simulink model "BothOptimized4"  (R2024b)
settings: Solver=FixedStepAuto  StartTime=0.0  StopTime=10.0  RelTol=1e-3  EnableMultiTasking=on
undefined symbols (not defined in the file or in its folder): samplingTime
settings Model: STM32="{\"DigitalPortWrite\":[{\"ID\":\"MicroMouseTemplate:84:3\"},{\"ID\":\"MicroMouseTemplate:84:4\"},{\"ID\":\"MicroMouseTemplate:84:5\"},{\"ID\":\"MicroMouseTemplate:84:6\"},{\"ID\":\"MicroMouseTemplate:84:7\"},{\"ID\":\"MicroMouseTemplate:84:8\"},{\"ID\":\"MicroMouseTemplate:84:9\"},{\"ID\":\"MicroMouseTemplate:84:10\"},{\"ID\":\"MicroMouseTemplate:160:19\"},{\"ID\":\"MicroMouseTemplate:2479:4\"},{\"ID\":\"MicroMouseTemplate:2479:6\"},{\"ID\":\"MicroMouseTemplate:2479:7\"},{\"ID\":\"MicroMouseTemplate:2479:8\"},{\"ID\":\"MicroMouseTemplate2:160:19\"},{\"ID\":\"MicroMouseTemplate2:2479:4\"},{\"ID\":\"MicroMouseTemplate2:2479:6\"},{\"ID\":\"MicroMouseTemplate2:2479:7\"},{\"ID\":\"MicroMouseTemplate2:2479:8\"},{\"ID\":\"MicroMouseTemplate2:84:3\"},{\"ID\":\"MicroMouseTemplate2:84:4\"},{\"ID\":\"MicroMouseTemplate2:84:5\"},{\"ID\":\"MicroMouseTemplate2:84:6\"},{\"ID\":\"MicroMouseTemplate2:84:7\"},{\"ID\":\"MicroMouseTemplate2:84:8\"},{\"ID\":\"MicroMouseTemplate2:84:9\"},{\"ID\":\"MicroMouseTemplate2:84:10\"},{\"ID\":\"MicroMouseTemplateTest:160:19\"},{\"ID\":\"MicroMouseTemplateTest:2479:4\"},{\"ID\":\"MicroMouseTemplateTest:2479:6\"},{\"ID\":\"MicroMouseTemplateTest:2479:7\"},{\"ID\":\"MicroMouseTemplateTest:2479:8\"},{\"ID\":\"MicroMouseTemplateTest:84:3\"},{\"ID\":\"MicroMouseTemplateTest:84:4\"},{\"ID\":\"MicroMouseTemplateTest:84:5\"},{\"ID\":\"MicroMouseTemplateTest:84:6\"},{\"ID\":\"MicroMouseTemplateTest:84:7\"},{\"ID\":\"MicroMouseTemplateTest:84:8\"},{\"ID\":\"MicroMouseTemplateTest:84:9\"},{\"ID\":\"MicroMouseTemplateTest:84:10\"},{\"ID\":\"MicroMouseTemplateTest2:160:19\"},{\"ID\":\"MicroMouseTemplateTest2:2479:4\"},{\"ID\":\"MicroMouseTemplateTest2:2479:6\"},{\"ID\":\"MicroMouseTemplateTest2:2479:7\"},{\"ID\":\"MicroMouseTemplateTest2:2479:8\"},{\"ID\":\"MicroMouseTemplateTest2:84:3\"},{\"ID\":\"MicroMouseTemplateTest2:84:4\"},{\"ID\":\"MicroMouseTemplateTest2:84:5\"},{\"ID\":\"MicroMouseTemplateTest2:84:6\"},{\"ID\":\"MicroMouseTemplateTest2:84:7\"},{\"ID\":\"MicroMouseTemplateTest2:84:8\"},{\"ID\":\"MicroMouseTemplateTest2:84:9\"},{\"ID\":\"MicroMouseTemplateTest2:84:10\"},{\"ID\":\"HalfOptimized:84:10\"},{\"ID\":\"HalfOptimized:84:9\"},{\"ID\":\"HalfOptimized:84:8\"},{\"ID\":\"HalfOptimized:84:7\"},{\"ID\":\"HalfOptimized:84:6\"},{\"ID\":\"HalfOptimized:84:5\"},{\"ID\":\"HalfOptimized:84:4\"},{\"ID\":\"HalfOptimized:84:3\"},{\"ID\":\"HalfOptimized:160:19\"},{\"ID\":\"HalfOptimized:2479:4\"},{\"ID\":\"HalfOptimized:2479:6\"},{\"ID\":\"HalfOptimized:2479:7\"},{\"ID\":\"HalfOptimized:2479:8\"},{\"ID\":\"HalfOptimized4:84:3\"},{\"ID\":\"HalfOptimized4:84:4\"},{\"ID\":\"HalfOptimized4:84:5\"},{\"ID\":\"HalfOptimized4:84:6\"},{\"ID\":\"HalfOptimized4:84:7\"},{\"ID\":\"HalfOptimized4:84:8\"},{\"ID\":\"HalfOptimized4:84:9\"},{\"ID\":\"HalfOptimized4:84:10\"},{\"ID\":\"HalfOptimized4:160:19\"},{\"ID\":\"HalfOptimized4:2479:4\"},{\"ID\":\"HalfOptimized4:2479:6\"},{\"ID\":\"HalfOptimized4:2479:7\"},{\"ID\":\"HalfOptimized4:2479:8\"},{\"ID\":\"LeftOptimized4:84:3\"},{\"ID\":\"LeftOptimized4:84:4\"},{\"ID\":\"LeftOptimized4:84:5\"},{\"ID\":\"LeftOptimized4:84:6\"},{\"ID\":\"LeftOptimized4:84:7\"},{\"ID\":\"LeftOptimized4:84:8\"},{\"ID\":\"LeftOptimized4:84:9\"},{\"ID\":\"LeftOptimized4:84:10\"},{\"ID\":\"LeftOptimized4:160:19\"},{\"ID\":\"LeftOptimized4:2479:4\"},{\"ID\":\"LeftOptimized4:2479:6\"},{\"ID\":\"LeftOptimized4:2479:7\"},{\"ID\":\"LeftOptimized4:2479:8\"}],\"PWMOutput\":[{\"ID\":\"MicroMouseTemplate:160:24\"},{\"ID\":\"MicroMouseTemplate:160:25\"},{\"ID\":\"MicroMouseTemplate2:160:24\"},{\"ID\":\"MicroMouseTemplate2:160:25\"},{\"ID\":\"MicroMouseTemplateTest:160:24\"},{\"ID\":\"MicroMouseTemplateTest:160:25\"},{\"ID\":\"MicroMouseTemplateTest2:160:24\"},{\"ID\":\"MicroMouseTemplateTest2:160:25\"},{\"ID\":\"HalfOptimized:160:24\"},{\"ID\":\"HalfOptimized:160:25\"},{\"ID\":\"HalfOptimized4:160:24\"},{\"ID\":\"HalfOptimized4:160:25\"},{\"ID\":\"LeftOptimized4:160:24\"},{\"ID\":\"LeftOptimized4:160:25\"}],\"AnalogInput\":[{\"ID\":\"MicroMouseTemplate:2357:1\"},{\"ID\":\"MicroMouseTemplate2:2357:1\"},{\"ID\":\"MicroMouseTemplateTest:2357:1\"},{\"ID\":\"MicroMouseTemplateTest2:2357:1\"},{\"ID\":\"HalfOptimized:2357:1\"},{\"ID\":\"HalfOptimized4:2357:1\"},{\"ID\":\"LeftOptimized4:2357:1\"}],\"DigitalPortRead\":[{\"ID\":\"MicroMouseTemplate:2483:3\"},{\"ID\":\"MicroMouseTemplate:2483:4\"},{\"ID\":\"MicroMouseTemplate2:2483:3\"},{\"ID\":\"MicroMouseTemplate2:2483:4\"},{\"ID\":\"MicroMouseTemplateTest:2483:3\"},{\"ID\":\"MicroMouseTemplateTest:2483:4\"},{\"ID\":\"MicroMouseTemplateTest2:2483:3\"},{\"ID\":\"MicroMouseTemplateTest2:2483:4\"},{\"ID\":\"HalfOptimized:2483:3\"},{\"ID\":\"HalfOptimized:2483:4\"},{\"ID\":\"HalfOptimized4:2483:3\"},{\"ID\":\"HalfOptimized4:2483:4\"},{\"ID\":\"LeftOptimized4:2483:3\"},{\"ID\":\"LeftOptimized4:2483:4\"}]}"  SimulationMode=external  ExtModeTrigDuration=10  Creator=JesseJabezArendse  LastModifiedBy=Nang'alelwa
settings SolverCC: AllowMultiTaskInputOutput=on  AutoInsertRateTranBlk=on  InsertRTBMode=Never (minimum delay)
settings OptimizationCC: EnhancedBackFolding=on  PassReuseOutputArgsAs=Individual arguments  StateBitsets=on  DataBitsets=on  ZeroExternalMemoryAtStartup=off  ZeroInternalMemoryAtStartup=off  NoFixptDivByZeroProtection=on  MaxStackSize=64  OptimizeBlockOrder=speed  DifferentSizesBufferReuse=on  EfficientTunableParamExpr=on
settings DebuggingCC: MultiTaskCondExecSysMsg=none  ParameterOverflowMsg=none  ParameterPrecisionLossMsg=none  ParameterTunabilityLossMsg=error
settings HardwareCC: ProdBitPerPointer=32  ProdBitPerSizeT=32  ProdBitPerPtrDiffT=32  ProdLargestAtomicInteger=Long  ProdLargestAtomicFloat=Double  ProdWordSize=32  ProdLongLongMode=on  ProdHWDeviceType=ARM Compatible->ARM Cortex  TargetBitPerPointer=64  TargetBitPerSizeT=64  TargetBitPerPtrDiffT=64  TargetLongLongMode=on  TargetIntDivRoundTo=Zero  TargetEndianess=LittleEndian  TargetWordSize=64  TargetHWDeviceType=MATLAB Host
settings ModelReferenceCC: EnableParallelModelReferenceBuilds=on  ParallelModelReferenceMATLABWorkerInit=Copy Base Workspace  SupportModelReferenceSimTargetCustomCode=on
settings SFSimCC: MATLABDynamicMemAlloc=off  SimHardwareAcceleration=native
settings RTWCC: Description=Embedded Coder  SystemTargetFile=ert.tlc  HardwareBoard=STM32L4xx Based  TLCOptions=-p0 -aInlineSetEventsForThisBaseRateFcn=TLC_FALSE -aSuppressMultiTaskScheduler=TLC_FALSE -aRateBasedStepFcn=1  TemplateMakefile=ert_default_tmf  Toolchain=GNU Tools for ARM Embedded Processors  CodeExecutionProfiling=on  CodeProfilingInstrumentation=coarse  GPUComputeCapability=3.5
settings RTWCC: CustomHeaderCode=|
  | #include "MicroMouseProgramming\Core\Inc\IMU.h"
  | #include "MicroMouseProgramming\Core\Inc\CustomWhile.h"
  | #include "MicroMouseProgramming\Core\Inc\Motors.h"
settings RTWCC: CustomInclude=|
  | MicroMouseProgramming\Core\Inc\
  | MicroMouseProgramming\Core\Src\
settings RTWCC: CustomSource=|
  | MicroMouseProgramming\Core\Src\IMU.c
  | MicroMouseProgramming\Core\Src\CustomWhile.c
  | MicroMouseProgramming\Core\Src\Motors.c
settings CodeAppCC: ForceParamTrailComments=on  IgnoreCustomStorageClasses=off  OperatorAnnotations=on  SimulinkDataObjDesc=on  SFDataObjDesc=on  InsertBlockDesc=on
settings ERTTargetCC: CodeReplacementLibrary=ARM Cortex-M  SupportNonFinite=off  SupportComplex=off  ExtModeTransport=3  ExtModeStaticAlloc=on  ExtModeStaticAllocSize=2048  ExtModeMexFile=ext_xcp  ExtModeIntrfLevel=Level2 - Open  InlinedParameterPlacement=Hierarchical  DynamicArrayContainerType=coder::array

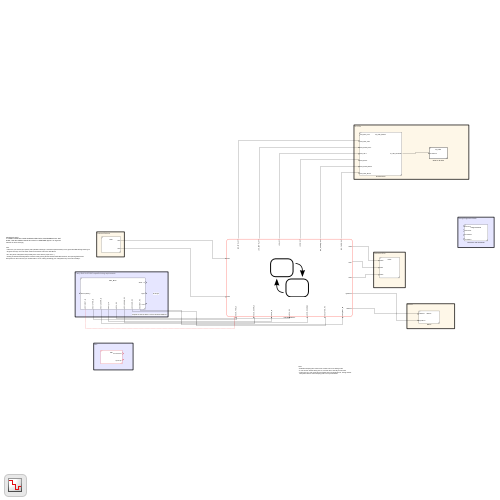
[thumbnail: Simulink's stored preview of the top-level diagram]
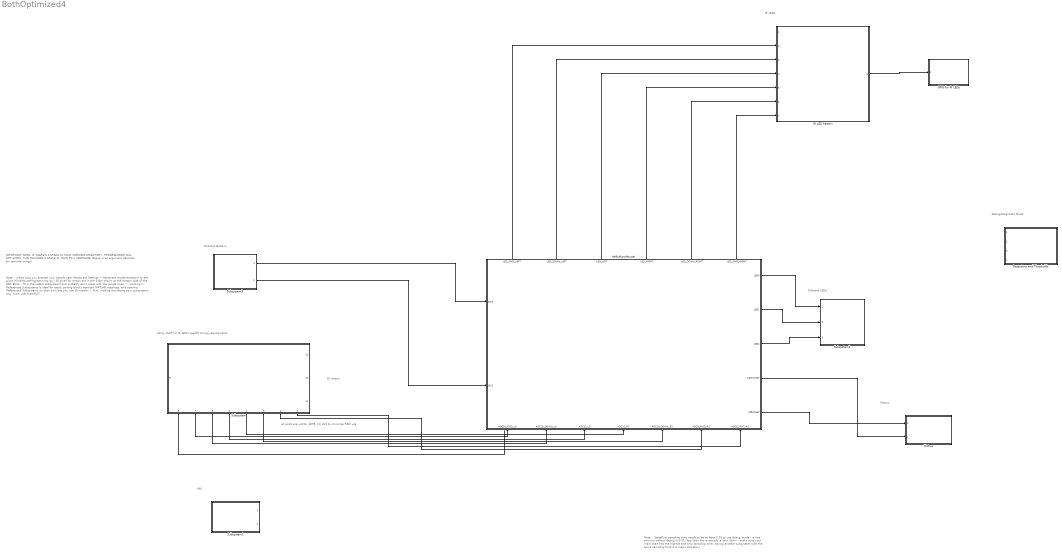
== system BothOptimized4 ==
  note: IMPORTANT NOTE:
      | IF THERE'S A SPACE IN YOUR WORKING DIRECTORY, PROGRAMMING WILL NOT WORK, THIS INCLUDES A SPACE IN YOUR PC's USERNAME (Space is an argument delimiter for terminal things)
  note: Note:
      | - make sure you entered your specifc path (Hardware Settings > Hardware Implementation) to the given MicroMouseProgramming.ioc
      | - All given 8x arrays are in the order shown at the bottom side of the ADC Block
      |
      | - fill in the yellow subsystems and probably don't mess with the purple ones :)
      | - working in Referenced Subsystems is ideal for easily porting blocks between MATLAB instances, and opening Referenced Subsystems on their own lets you use Simulation > Run, making simulating your subsystems way more user friendly!!!
  note: 8x arrays
  note: all ports are uint16, 4095 == 3V3 to minimize RAM use
  note: IMU
  note: Note:
      | - Stateflow sampling time needs to be at least 0.05 to use debug mode
      | - a nice amount without debug is 0.01, less than this is actually a slow down
      | - make sure your main chart has the highest and only sampling time, having another
      | subsystem with the same sampling time is a major slowdown
  note: Fancy Stuff for IR ADCs specific timing requirements
  note: IR LEDs
  note: Motors
  note: Onboard Buttons
  note: Onboard LEDs
  note: Debug/Diagnostic Mode
  Detections and Thresholds : Subsystem  ReferencedSubsystem=DiagnosticMode
  GPIO for IR LEDs : Subsystem  TreatAsAtomicUnit=on  SystemSampleTime=samplingTime  ReferencedSubsystem=IR_LEDs
  HelloMicroMouse! : Stateflow chart  TreatAsAtomicUnit=on
      settings: PortSchema="{\"entries\":[{\"content\":{\"sides\":[{\"content\":{\"connectorIds\":[\"In9\",\"In8\"]},\"type\":\"ConnectorPlacement.EquallySpacedRectSide\",\"uuid\":\"f52daa4f-6374-42e5-9ef1-0ccc99d09b58\"},{\"content\":{\"connectorIds\":[\"Out11\",\"Out5\",\"Out6\",\"Out2\",\"Out1\"],\"side\":\"RIGHT\"},\"type\":\"ConnectorPlacement.EquallySpacedRectSide\",\"uuid\":\"94b478cc-4dde-45c7-a588-77cf2b43cdb7\"},{\"content\":{\"connectorIds\":[\"Out3\",\"Out4\",\"Out7\",\"Out8\",\"Out9\",\"Out10\"],\"side\":\"TOP\"},\"type\":\"ConnectorPlacement.EquallySpacedRectSide\",\"uuid\":\"afff2079-ea5c-423e-9722-09c3bbce433b\"},{\"content\":{\"connectorIds\":[\"In1\",\"In2\",\"In3\",\"In4\",\"In5\",\"In6\",\"In7\"],\"side\":\"BOTTOM\"},\"type\":\"ConnectorPlacement.EquallySpacedRectSide\",\"uuid\":\"94e93a1d-795d-41a3-b2d8-d520b2bf47ef\"}]},\"type\":\"ConnectorPlacement.EquallySpacedConnector\",\"uuid\":\"d4d35636-54af-48ac-af70-d56caef5e090\"}],\"packageUris\":[\"http://schema.mathworks.com/mf0/Connector/R2020b\"],\"version\":\"1.0\"}"
  IR LED Pattern : Subsystem  ReferencedSubsystem=IR_LED_Pattern
  Motors : Subsystem  ReferencedSubsystem=Motors
      settings: PortSchema="{\"entries\":[{\"content\":{\"sides\":[{\"content\":{\"connectorIds\":[\"In2\",\"In1\"]},\"type\":\"ConnectorPlacement.EquallySpacedRectSide\",\"uuid\":\"b3741f01-871a-479c-9206-f0581f668097\"},{\"content\":{\"side\":\"RIGHT\"},\"type\":\"ConnectorPlacement.EquallySpacedRectSide\",\"uuid\":\"4e24163a-f10e-40fa-a35f-86add3e4876d\"},{\"content\":{\"side\":\"TOP\"},\"type\":\"ConnectorPlacement.EquallySpacedRectSide\",\"uuid\":\"20b900cb-8f31-42f3-9ac1-0d679ccd8bc0\"}]},\"type\":\"ConnectorPlacement.EquallySpacedConnector\",\"uuid\":\"90358f46-f7a9-48cf-9149-c68081c17f53\"}],\"packageUris\":[\"http://schema.mathworks.com/mf0/Connector/R2020b\"],\"version\":\"1.0\"}"
  Subsystem : Subsystem  ReferencedSubsystem=ADC_Block
      settings: PortSchema="{\"entries\":[{\"content\":{\"sides\":[{\"content\":{},\"type\":\"ConnectorPlacement.EquallySpacedRectSide\",\"uuid\":\"be6b81d5-7a49-4e34-b35f-0c07892094fc\"},{\"content\":{\"connectorIds\":[\"Out1\",\"Out2\",\"Out3\",\"Out4\",\"Out5\",\"Out6\",\"Out7\",\"Out8\"],\"side\":\"RIGHT\"},\"type\":\"ConnectorPlacement.EquallySpacedRectSide\",\"uuid\":\"5e22590a-b7c0-4c63-8de4-8d81fd6c3849\"},{\"content\":{\"connectorIds\":[\"Out12\",\"Out10\",\"Out11\"],\"side\":\"TOP\"},\"type\":\"ConnectorPlacement.EquallySpacedRectSide\",\"uuid\":\"da97636e-cea0-4a10-8fe5-d807f9ee999f\"},{\"content\":{\"connectorIds\":[\"Out9\"],\"side\":\"BOTTOM\"},\"type\":\"ConnectorPlacement.EquallySpacedRectSide\",\"uuid\":\"a593d780-81a8-4730-a8bc-2bbf356cafe4\"}]},\"type\":\"ConnectorPlacement.EquallySpacedConnector\",\"uuid\":\"0bcac921-e51a-4437-9183-315712d0a8c2\"}],\"packageUris\":[\"http://schema.mathworks.com/mf0/Connector/R2020b\"],\"version\":\"1.0\"}"
  Subsystem1 : Subsystem  ReferencedSubsystem=IMU
  Subsystem2 : Subsystem  ReferencedSubsystem=LEDs
  Subsystem3 : Subsystem  ReferencedSubsystem=SWs
  wires:
  HelloMicroMouse!/2(rightWheel) -> Motors/1
  HelloMicroMouse!/1(leftWheel) -> Motors/2
  IR LED Pattern/1 -> GPIO for IR LEDs/1
  Subsystem3/1 -> HelloMicroMouse!/9(SW1)
  Subsystem3/2 -> HelloMicroMouse!/8(SW2)
  HelloMicroMouse!/11(LED0) -> Subsystem2/1
  Subsystem/8 -> ?
  Subsystem/7 -> HelloMicroMouse!/1(ADC14_FWD_LS)
  Subsystem/6 -> HelloMicroMouse!/2(ADC13_DOWN_LS)
  Subsystem/5 -> HelloMicroMouse!/3(ADC12_LS)
  Subsystem/4 -> HelloMicroMouse!/4(ADC11_RS)
  Subsystem/3 -> HelloMicroMouse!/5(ADC10_DOWN_RS)
  Subsystem/2 -> HelloMicroMouse!/6(ADC9_FWD_RS)
  Subsystem/1 -> HelloMicroMouse!/7(ADC8_MOT_RS)
  HelloMicroMouse!/5(LED1) -> Subsystem2/2
  HelloMicroMouse!/6(LED2) -> Subsystem2/3
  HelloMicroMouse!/10(LED_FWD_RIGHT) -> IR LED Pattern/7
  HelloMicroMouse!/9(LED_DOWN_RIGHT) -> IR LED Pattern/6
  HelloMicroMouse!/8(LED_RIGHT) -> IR LED Pattern/5
  HelloMicroMouse!/7(LED_LEFT) -> IR LED Pattern/4
  HelloMicroMouse!/4(LED_DOWN_LEFT) -> IR LED Pattern/3
  HelloMicroMouse!/3(LED_FWD_LEFT) -> IR LED Pattern/2

== stateflow chart BothOptimized4/HelloMicroMouse! ==
  state ButtonPressed6 [commented out]
    entry:
    LED0 = false;
    LED1 = false;
    LED2 = false;
    state Turning_Right_Adjustment [commented out]
      entry:
      LED2 = true;
      leftWheel = 75;
      rightWheel = 70;
      exit:
      leftWheel = 0;
      LED2 = false;
    state Forward [commented out]
      entry:
      LED1 = true;
      % if abs(ADC13_DOWN_LS - ADC10_DOWN_RS) > down_error
      %    error = true;
      %    check = max(ADC13_DOWN_LS - thresh_down_l, ADC10_DOWN_RS - thresh_down_r)
      %end
      leftWheel = normal_speed_LEFT;
      rightWheel = normal_speed_RIGHT;
      exit:
      LED1 = false;
      % during:
      % curr_d_left = ADC13_DOWN_LS;
      % curr_d_right = ADC10_DOWN_RS;
      % if abs(curr_d_left - curr_d_right) > down_error
      %     error = true;
      %    check = max((curr_d_left - thresh_down_l)*0.8, curr_d_right - thresh_down_r)
      % end
    state Turning_Left_Adjustment [commented out]
      entry:
      LED0 = true;
      rightWheel = 75;
      leftWheel = 70;
      exit:
      rightWheel = 0;
      LED0 = false;
    (default) -> ButtonPressed6.Forward [commented out]
    ButtonPressed6.Forward -> ButtonPressed6.Turning_Right_Adjustment [commented out] : [(ADC13_DOWN_LS > thresh_DOWN_LEFT) ]
    ButtonPressed6.Turning_Right_Adjustment -> ButtonPressed6.Forward [commented out] : after(0.2, sec)
    ButtonPressed6.Forward -> ButtonPressed6.Turning_Left_Adjustment [commented out] : [(ADC10_DOWN_RS > thresh_DOWN_RIGHT) ]
    ButtonPressed6.Turning_Left_Adjustment -> ButtonPressed6.Forward [commented out] : after(0.2, sec)
  state Turns1
    entry:
    solved = 0
    LED0 = false;
    LED1 = false;
    LED2 = false;
    R = 1;
    S = 2;
    L = 3;
    B = 4;
    stop = 0
    state TurnLeftToLeft1
      entry:
      leftWheel = -75;
      rightWheel = 75;
    state CheckLeftWall1
      entry:
      leftWheel = 0;
      rightWheel = 0;
      if (ADC14_FWD_LS >0.85* init_FWD_LEFT &&  ADC9_FWD_RS >0.85* init_FWD_RIGHT)
      LED1 = false;
      else
      SolvedAlgorithm(index) = L;
      index = index +1;
      stop = 1
      LED1 = true;
      end
    state MoveCentre
      entry:
      leftWheel = 75;
      rightWheel = 75;
    state CheckStraightWall
      entry:
      leftWheel = 0;
      rightWheel = 0;
      if (ADC14_FWD_LS >0.85* init_FWD_LEFT &&  ADC9_FWD_RS >0.8* init_FWD_RIGHT)
      LED1 = false;
      else
      SolvedAlgorithm(index) = S;
      index = index +1;
      stop = 1;
      LED1 = true;
      end
    state TurnRightToStraight
      entry:
      leftWheel = 75;
      rightWheel = -75;
    state CheckLeftWall
      entry:
      leftWheel = 0;
      rightWheel = 0;
      if (ADC14_FWD_LS >0.80* init_FWD_LEFT &&  ADC9_FWD_RS >0.85* init_FWD_RIGHT)
      LED1 = false;
      else
      SolvedAlgorithm(index) = R;
      index = index +1;
      stop = 1
      LED1 = true;
      end
    state TurnRightToRight
      entry:
      leftWheel = 75;
      rightWheel = -75;
    state CheckWallBack
      entry:
      leftWheel = 0;
      rightWheel = 0;
      during:
      if (ADC14_FWD_LS >0.85* init_FWD_LEFT &&  ADC9_FWD_RS >0.87* init_FWD_RIGHT)
      LED1 = false;
      else
      SolvedAlgorithm(index) = B;
      index = index +1;
      stop = 1
      LED1 = true;
      end
    state TurnLeftToBack
      entry:
      leftWheel = 75;
      rightWheel = -75;
    (default) -> Turns1.MoveCentre
    Turns1.CheckWallBack -> TurnLeftToLeft1 : [SW2]
    TurnLeftToLeft1 -> CheckLeftWall1 : after(1.2, sec)
    Turns1.MoveCentre -> TurnLeftToLeft1 : after(0.4,sec)
    CheckLeftWall1 -> TurnRightToStraight : after(1.2,sec)
    TurnRightToStraight -> Turns1.CheckStraightWall : after(1.2,sec)
    Turns1.CheckStraightWall -> Turns1.TurnRightToRight : after(1.1,sec)
    Turns1.TurnRightToRight -> Turns1.CheckLeftWall : after(1.2,sec)
    Turns1.CheckLeftWall -> Turns1.TurnLeftToBack : after(1.2,sec)
    Turns1.TurnLeftToBack -> Turns1.CheckWallBack : after(1.2 ,sec)
  state ButtonPressed8 [commented out]
    entry:
    LED0 = false;
    LED1 = false;
    LED2 = false;
    state Driving [commented out]
      % State: Waiting
      entry:
      timer = 0;
      during:
      timer = timer + 1;
      % Transition Condition
      [timer >= 100]
      state Straight [commented out]
        entry:
        leftWheel = 75;
        rightWheel = 75;
        LED0 =false;
        LED2 = false;
        LED1 = false;
      state TurnLeft [commented out]
        entry:
        leftWheel = 75;
        rightWheel = 85;
        LED0 = true;
        LED2 = false;
        LED1 = false;
      state TurnRight [commented out]
        entry:
        rightWheel = 75;
        leftWheel = 85;
        LED2 = true;
        LED0 =false;
        LED1 =false;
      (default) -> Straight [commented out]
      Straight -> ButtonPressed8.Driving.TurnRight [commented out] : [ADC13_DOWN_LS>thresh_DOWN_LEFT]
      Straight -> ButtonPressed8.Driving.TurnLeft [commented out] : [ADC10_DOWN_RS > thresh_DOWN_RIGHT]
      ButtonPressed8.Driving.TurnLeft -> Straight [commented out] : [ADC10_DOWN_RS < thresh_DOWN_RIGHT && ADC13_DOWN_LS<thresh_DOWN_LEFT ]
      ButtonPressed8.Driving.TurnRight -> Straight [commented out] : [ADC10_DOWN_RS < thresh_DOWN_RIGHT && ADC13_DOWN_LS<thresh_DOWN_LEFT]
      ButtonPressed8.Driving.TurnRight -> ButtonPressed8.Driving.TurnLeft [commented out] : [ADC10_DOWN_RS > thresh_DOWN_RIGHT]
      ButtonPressed8.Driving.TurnLeft -> ButtonPressed8.Driving.TurnRight [commented out] : [ADC13_DOWN_LS>thresh_DOWN_LEFT]
    state FrontDetection [commented out]
      entry:
      leftWheel = 0;
      rightWheel = 0;
      LED0 =false;
      LED1 = true;
      LED2 = false;
    state CrossDetection [commented out]
      entry:
      flag = 1;
      leftWheel = 0;
      rightWheel = 0;
      LED0 =true;
      LED1 = true;
      LED2 = true;
    (default) -> Driving [commented out]
    Driving -> FrontDetection [commented out] : [averageFront > frontThreshold]
    FrontDetection -> Driving [commented out] : [averageFront< frontThreshold]
    Driving -> CrossDetection [commented out] : [averageDown < crossThreshold && timer >= 100]
    CrossDetection -> Driving [commented out] : [after(1000, msec)]{LED1 = false;}
  state Calibration_Down3 [commented out]
    entry:
    LED1 = true
    LED_FWD_LEFT = true;
    LED_FWD_RIGHT = true;
    LED_DOWN_RIGHT = true;
    LED_DOWN_LEFT = true;
    rightWheel = 75;
    leftWheel = -75;
    DOWN_R_DARK = ADC10_DOWN_RS;
    DOWN_L_DARK = ADC13_DOWN_LS;
    DOWN_R_LIGHT = ADC10_DOWN_RS;
    DOWN_L_LIGHT = ADC13_DOWN_LS;
    during:
    DOWN_R_DARK = min(DOWN_R_DARK, ADC10_DOWN_RS);
    DOWN_L_DARK = min(DOWN_L_DARK, ADC13_DOWN_LS);
    DOWN_R_LIGHT = max(DOWN_R_LIGHT, ADC10_DOWN_RS);
    DOWN_L_LIGHT = max(DOWN_L_LIGHT, ADC13_DOWN_LS);
  state Calibration_Forward3 [commented out]
    entry:
    LED1 = true;
    LED_FWD_LEFT = true;
    LED_FWD_RIGHT = true;
    LED_DOWN_RIGHT = true;
    LED_DOWN_LEFT = true;
    counter = 0
    sum_FWD_LEFT = 0;
    sum_FWD_RIGHT = 0;
    during:
    % Collect ADC values for averaging
    if counter < 100
    sum_FWD_LEFT = sum_FWD_LEFT + ADC14_FWD_LS;
    sum_FWD_RIGHT = sum_FWD_RIGHT + ADC9_FWD_RS;
    counter = counter + 1;
    else
    % Once 10 samples are collected, calculate the average
    avg_FWD_LEFT = sum_FWD_LEFT / counter;
    avg_FWD_RIGHT = sum_FWD_RIGHT / counter;
    % Use the averages for calibration or further processing
    init_FWD_LEFT = avg_FWD_LEFT;
    init_FWD_RIGHT = avg_FWD_RIGHT;
    end
  state Stop8 [commented out]
    entry:
    LED0 = false;
    LED2 = false;
    leftWheel = 0;
    rightWheel = 0;
    during:
    LED1 = ~LED1;
  state Ready4 [commented out]
    entry:
    rightWheel = 0;
    leftWheel = 0;
    LED2 = true;
    LED0 = true;
    %thresh_DOWN_RIGHT = init_DOWN_R_DARK*1.5
    %thresh_DOWN_LEFT = init_DOWN_L_DARK*1.5
    thresh_DOWN_RIGHT = (DOWN_R_LIGHT + DOWN_R_DARK)*0.5;
    thresh_DOWN_LEFT = (DOWN_L_LIGHT + DOWN_L_DARK)*0.5;
    % down_error = abs(dark_val_r - dark_val_l);
    normal_speed_LEFT = 75;
    normal_speed_RIGHT = 75;
  state WaitUntilButtonPressed10 [commented out]
    entry:
    LED_MOT_LEFT = false;
    LED_MOT_RIGHT = false;
    LED_FWD_LEFT = false;
    LED_FWD_RIGHT = false;
    LED_LEFT = false;
    LED_RIGHT = false;
    LED_DOWN_RIGHT = false;
    LED_DOWN_LEFT = false;
    during:
    LED1 = ~LED1;
  state Turns [commented out]
    entry:
    solved = 0
    LED0 = false;
    LED1 = false;
    LED2 = false;
    R = 1;
    S = 2;
    L = 3;
    B = 4;
    state TurnRightToRight [commented out]
      entry:
      leftWheel = 75;
      rightWheel = -75;
    state CheckRightWall [commented out]
      entry:
      leftWheel = 0;
      rightWheel = 0;
      if (ADC14_FWD_LS >0.85* init_FWD_LEFT &&  ADC9_FWD_RS >0.85* init_FWD_RIGHT)
      LED1 = false;
      else
      SolvedAlgorithm(index) = R;
      index = index +1;
      LED1 = true;
      end
    state MoveCentre [commented out]
      entry:
      leftWheel = 75;
      rightWheel = 75;
    state CheckStraightWall [commented out]
      entry:
      leftWheel = 0;
      rightWheel = 0;
      if (ADC14_FWD_LS >0.85* init_FWD_LEFT &&  ADC9_FWD_RS >0.85* init_FWD_RIGHT)
      LED1 = false;
      else
      SolvedAlgorithm(index) = S;
      index = index +1;
      LED1 = true;
      end
    state TurnLeftToStraight [commented out]
      entry:
      leftWheel = -75;
      rightWheel = 75;
    state CheckLeftWall [commented out]
      entry:
      leftWheel = 0;
      rightWheel = 0;
      if (ADC14_FWD_LS >0.85* init_FWD_LEFT &&  ADC9_FWD_RS >0.85* init_FWD_RIGHT)
      LED1 = false;
      else
      SolvedAlgorithm(index) = L;
      index = index +1;
      LED1 = true;
      end
    state TurnLeftToLeft [commented out]
      entry:
      leftWheel = -75;
      rightWheel = 75;
    state CheckWallBack [commented out]
      entry:
      leftWheel = 0;
      rightWheel = 0;
      during:
      if (ADC14_FWD_LS >0.85* init_FWD_LEFT &&  ADC9_FWD_RS >0.85* init_FWD_RIGHT)
      LED1 = false;
      else
      SolvedAlgorithm(index) = B;
      index = index +1;
      LED1 = true;
      end
    state TurnLeftToBack [commented out]
      entry:
      leftWheel = -75;
      rightWheel = 75;
    (default) -> Turns.MoveCentre [commented out]
    Turns.CheckWallBack -> Turns.TurnRightToRight [commented out] : [SW2]
    Turns.TurnRightToRight -> CheckRightWall [commented out] : after(1.05, sec)
    Turns.MoveCentre -> Turns.TurnRightToRight [commented out] : after(0.4,sec)
    CheckRightWall -> TurnLeftToStraight [commented out] : after(1.1,sec)
    TurnLeftToStraight -> Turns.CheckStraightWall [commented out] : after(1.2,sec)
    Turns.CheckStraightWall -> TurnLeftToLeft [commented out] : after(1.1,sec)
    TurnLeftToLeft -> Turns.CheckLeftWall [commented out] : after(1.2,sec)
    Turns.CheckLeftWall -> Turns.TurnLeftToBack [commented out] : after(1.1,sec)
    Turns.TurnLeftToBack -> Turns.CheckWallBack [commented out] : after(1.2 ,sec)
  state Placeholder2
    entry:
    index = 1;
    leftWheel = 0;
    rightWheel = 0;
    solved = 1;
    during:
    LED1=~LED1;
  state ButtonPressed7 [commented out]
    entry:
    LED1 = false;
    LED0 = false;
    LED2 = false;
    state Check_Front [commented out]
      entry:
      leftWheel = 0;
      rightWheel = 0;
      LED1 = ~LED1;
      LED0 = false;
      LED2 = ~LED2;
      during:
      LED1 = ~LED1;
      LED0 = false;
      LED2 = ~LED2;
    state Reverse [commented out]
      entry:
      leftWheel = -75;
      rightWheel = -75;
    state Turn_Around [commented out]
      entry:
      leftWheel = -motor_speed_left;
      rightWheel = motor_speed_right;
      during:
      LED1 = ~LED1;
      LED0 = ~LED0;
      LED2 = ~LED2;
    state Off_Left [commented out]
      entry:
      LED0 = true;
      leftWheel = 75;
      rightWheel = 70;
      exit:
      leftWheel = 0;
      LED0 = false;
    state Forward [commented out]
      entry:
      LED1 = false;
      LED0 = false;
      LED2 = false;
      LED_FWD_RIGHT = 1;
      LED_FWD_LEFT = 1;
      LED_RIGHT = 0;
      LED_LEFT = 0;
      leftWheel = motor_speed_left;
      rightWheel = motor_speed_right;
    state Off_Right [commented out]
      entry:
      LED2 = true;
      rightWheel = 75;
      leftWheel = 70;
      exit:
      rightWheel = 0;
      LED2 = false;
    state Check_Right [commented out]
      entry:
      LED1 = true;
      %ambient_RIGHT = ADC11_RS;
      %ambient_LEFT = ADC12_LS;
      LED_FWD_RIGHT = 0;
      LED_FWD_LEFT = 0;
      LED_RIGHT = 1;
      LED_LEFT = 1;
      leftWheel = 0;
      rightWheel = 0;
    state Turn_Right [commented out]
      entry:
      leftWheel = motor_speed_left;
      rightWheel = -motor_speed_right;
      LED_FWD_RIGHT = 1;
      LED_FWD_LEFT = 1;
      LED_RIGHT = 0;
      LED_LEFT = 0;
      LED1 = true;
      LED0 = true;
      LED2 = true;
    state Checking [commented out]
      during:
      LED1 = ~LED1
      %right_dif = abs(ADC11_RS - ambient_RIGHT);
      %left_dif = abs(ADC12_LS - ambient_LEFT);
      exit:
      LED1 = true;
    state Waiting [commented out]
      entry:
      leftWheel = motor_speed_left;
      rightWheel = motor_speed_right;
      LED1 = true;
      LED0 = true;
      LED2 = true;
    Turn_Around -> (junction 373) [commented out] : after(1.2, sec)
    (junction 373) -> Check_Front [commented out] : [ADC10_DOWN_RS >= thresh_down_r*1.15 && ADC10_DOWN_RS > thresh_down_r*1.15]
    Reverse -> Turn_Around [commented out] : [ADC13_DOWN_LS <= dark_val_l*1.15 && ADC10_DOWN_RS <= dark_val_r*1.15]
    Check_Front -> Turn_Around [commented out] : [ADC14_FWD_LS > init_FWD_LEFT || ADC9_FWD_RS > init_FWD_RIGHT]
    Reverse -> Turn_Around [commented out] : after(1,sec)
    ButtonPressed7.Forward -> Reverse [commented out] : [ADC14_FWD_LS > init_FWD_LEFT &&  ADC9_FWD_RS > init_FWD_RIGHT]
    Check_Front -> ButtonPressed7.Forward [commented out] : [ADC14_FWD_LS <= init_FWD_LEFT ||  ADC9_FWD_RS <= init_FWD_RIGHT]
    (junction 368) -> Off_Left [commented out] : [(ADC13_DOWN_LS - thresh_down_l) > (ADC10_DOWN_RS - thresh_down_r)]
    (default) -> ButtonPressed7.Forward [commented out]
    ButtonPressed7.Forward -> Off_Left [commented out] : [ADC13_DOWN_LS > thresh_down_l]
    Off_Left -> ButtonPressed7.Forward [commented out] : after(0.2, sec)
    ButtonPressed7.Forward -> Off_Right [commented out] : [ADC10_DOWN_RS > thresh_down_r]
    Off_Right -> ButtonPressed7.Forward [commented out] : after(0.2, sec)
    ButtonPressed7.Forward -> Check_Right [commented out] : [ADC13_DOWN_LS <= dark_val_l*1.15 && ADC10_DOWN_RS <= dark_val_r*1.15]
    (junction 364) -> ButtonPressed7.Forward [commented out] : [ADC10_DOWN_RS <= thresh_down_r*1.15 && ADC13_DOWN_LS <= thresh_down_l*1.15]
    ButtonPressed7.Forward -> (junction 368) [commented out] : [ADC13_DOWN_LS > thresh_down_l && ADC10_DOWN_RS > thresh_down_r]
    (junction 368) -> Off_Right [commented out] : [(ADC13_DOWN_LS - thresh_down_l) < (ADC10_DOWN_RS - thresh_down_r)]
    Turn_Right -> (junction 364) [commented out] : after(0.8, sec)
    Check_Right -> Checking [commented out] : after(0.2, sec)
    Waiting -> Turn_Right [commented out] : after(0.5, sec)
    Checking -> Waiting [commented out] : after(0.3, sec)
  state Stop7 [commented out]
    entry:
    LED_FWD_LEFT = 0;
    LED_FWD_RIGHT = 0;
    LED_LEFT = 1;
    LED_RIGHT = 1;
    LED0 = false;
    LED2 = false;
    leftWheel = 0;
    rightWheel = 0;
    during:
    if ADC11_RS >= thresh_RIGHT;
    LED0 = true;
    else
    LED0 = false;
    end
    if ADC12_LS >= thresh_LEFT;
    LED2 = true;
    else
    LED2 = false;
    end
    exit:
    LED0 = false;
    LED2 = false;
  state Side_Calibration [commented out]
    entry:
    lr_count = 0;
    LED1 = true;
    LED_LEFT = 1;
    LED_RIGHT = 1;
    LED_FWD_LEFT = 0;
    LED_FWD_RIGHT = 0;
    rightWheel = 75;
    leftWheel = -75;
    dark_val_r=ADC10_DOWN_RS;
    dark_val_l=ADC13_DOWN_LS;
    light_val_r = ADC10_DOWN_RS;
    light_val_l = ADC13_DOWN_LS;
    during:
    lr_count = lr_count + 1
    dark_val_r = min(dark_val_r, ADC10_DOWN_RS);
    dark_val_l = min(dark_val_l, ADC13_DOWN_LS);
    light_val_r = max(light_val_r, ADC10_DOWN_RS);
    light_val_l = max(light_val_l, ADC13_DOWN_LS);
    %dark_val_mot_r = min(dark_val_mot_r, MOT_RS);
    %dark_val_mot_l = min(dark_val_mot_l, MOT_LS);
    %light_val_mot_r = max(light_val_mot_r, MOT_RS);
    %light_val_mot_l = max(light_val_mot_l, MOT_LS);
    init_RIGHT = max(init_RIGHT, ADC11_RS);
    init_LEFT = max(init_LEFT, ADC12_LS);
  state Forward_Calibration [commented out]
    entry:
    fwd_count = 0;
    LED2 = true
    rightWheel = 75;
    leftWheel = -75;
    init_FWD_LEFT = ADC14_FWD_LS;
    init_FWD_RIGHT = ADC9_FWD_RS;
    during:
    fwd_count = fwd_count + 1;
    dark_val_r = min(dark_val_r, ADC10_DOWN_RS);
    dark_val_l = min(dark_val_l, ADC13_DOWN_LS);
    light_val_r = max(light_val_r, ADC10_DOWN_RS);
    light_val_l = max(light_val_l, ADC13_DOWN_LS);
    %dark_val_mot_r = min(dark_val_mot_r, MOT_RS);
    %dark_val_mot_l = min(dark_val_mot_l, MOT_LS);
    %light_val_mot_r = max(light_val_mot_r, MOT_RS);
    %light_val_mot_l = max(light_val_mot_l, MOT_LS);
    init_FWD_LEFT = max(init_FWD_LEFT, ADC14_FWD_LS);
    init_FWD_RIGHT = max(init_FWD_RIGHT, ADC9_FWD_RS);
    %ambient_LEFT = ambient_LEFT + ADC12_LS;
    %ambient_RIGHT = ambient_RIGHT + ADC11_RS;
  state Ready_To_Go2 [commented out]
    entry:
    rightWheel = 0;
    leftWheel = 0;
    LED2 = true;
    LED0 = true;
    init_LEFT = init_LEFT;
    init_RIGHT = init_RIGHT;
    %ambient_RIGHT = ambient_RIGHT/lr_count;
    %ambient_LEFT = ambient_LEFT/fwd_count;
    %thresh_RIGHT = abs(init_RIGHT - ambient_RIGHT);
    %thresh_LEFT = abs(init_LEFT - ambient_LEFT);
    thresh_RIGHT = init_RIGHT*0.7;
    thresh_LEFT = init_LEFT*0.7;
    %init_FWD_LEFT = init_FWD_LEFT / fwd_count;
    %init_FWD_RIGHT = init_FWD_RIGHT / fwd_count;
    init_FWD_LEFT = init_FWD_LEFT*0.8;
    init_FWD_RIGHT = init_FWD_RIGHT*0.8;
    thresh_down_r = (light_val_r + dark_val_r)*0.5;
    thresh_down_l = (light_val_l + dark_val_l)*0.5;
    %thresh_down_mot_r = (light_val_mot_r + dark_val_mot_r)*0.5;
    %thresh_down_mot_l = (light_val_mot_l + dark_val_mot_l)*0.5;
    motor_speed_left = 75;
    motor_speed_right = 75;
  state Ready_To_Go [commented out]
    entry:
    LED_DOWN_LEFT = 1
    LED_DOWN_RIGHT = 1
    LED_LEFT = 1;
    LED_RIGHT = 1;
    LED_FWD_LEFT = 0;
    LED_FWD_RIGHT = 0;
    init_RIGHT = ADC11_RS;
    init_LEFT = ADC12_LS;
    during:
    LED1 = ~LED1;
  state WaitUntilButtonPressed9 [commented out]
    during:
    LED0 = ~LED0;
    exit:
    LED0 = false;
    LED2 = false;
  state Calibration_Forward1
    entry:
    LED0 = false;
    LED1 = true;
    LED2 = false
    LED_LEFT = false;
    LED_RIGHT = false;
    LED_FWD_LEFT = true;
    LED_FWD_RIGHT = true;
    LED_DOWN_RIGHT = true;
    LED_DOWN_LEFT = true;
    counter = 0
    sum_FWD_LEFT = 0;
    sum_FWD_RIGHT = 0;
    during:
    if counter < 8000
    sum_FWD_LEFT = sum_FWD_LEFT + ADC14_FWD_LS;
    sum_FWD_RIGHT = sum_FWD_RIGHT + ADC9_FWD_RS;
    counter = counter + 1;
    end
    exit:
    avg_FWD_LEFT = sum_FWD_LEFT / counter;
    avg_FWD_RIGHT = sum_FWD_RIGHT / counter;
    init_FWD_LEFT = avg_FWD_LEFT;
    init_FWD_RIGHT = avg_FWD_RIGHT;
    LED1 = false
  state LineFollowing
    entry:
    LED0 = false;
    LED1 = false;
    LED2 = false;
    LED_LEFT = false;
    LED_RIGHT = false;
    LED_FWD_LEFT = true;
    LED_FWD_RIGHT = true;
    LED_DOWN_RIGHT = true;
    LED_DOWN_LEFT = true;
    exit:
    LED0 = false;
    LED1 = false;
    LED2 = false;
    state Forward
      entry:
      LED1 = true;
      leftWheel = 80;
      rightWheel = 80;
      exit:
      LED1 = false;
    state Turning_Right_Adjustment
      entry:
      LED2 = true;
      leftWheel = 80;
      rightWheel = 70;
      exit:
      leftWheel = 0;
      LED2 = false;
    state Turning_Left_Adjustment
      entry:
      LED0 = true;
      rightWheel = 80;
      leftWheel = 70;
      exit:
      rightWheel = 0;
      LED0 = false;
    (default) -> LineFollowing.Forward
    LineFollowing.Forward -> LineFollowing.Turning_Right_Adjustment [order 1] : [(ADC10_DOWN_RS >ADC13_DOWN_LS )  ]
    LineFollowing.Turning_Right_Adjustment -> LineFollowing.Forward
    LineFollowing.Forward -> LineFollowing.Turning_Left_Adjustment [order 2] : [(ADC10_DOWN_RS < ADC13_DOWN_LS ) ]
    LineFollowing.Turning_Left_Adjustment -> LineFollowing.Forward
  state Calibration_Left_and_Right
    entry:
    LED0 = true;
    LED1 = false;
    LED2 = false
    LED_LEFT = true;
    LED_RIGHT = true;
    LED_FWD_LEFT = false;
    LED_FWD_RIGHT = false;
    LED_DOWN_RIGHT = false;
    LED_DOWN_LEFT = false;
    counter2 = 0
    sum_LEFT = 0;
    sum_RIGHT = 0;
    during:
    if counter2 < 8000
    sum_LEFT = sum_LEFT + ADC12_LS;
    sum_RIGHT = sum_RIGHT + ADC11_RS;
    counter2 = counter2 + 1;
    end
    exit:
    % Once 10 samples are collected, calculate the average
    avg_LEFT = sum_LEFT / counter2;
    avg_RIGHT = sum_RIGHT / counter2;
    % Use the averages for calibration or further processing
    init_LEFT = avg_LEFT;
    init_RIGHT = avg_RIGHT;
    end
    exit:
    LED0 = false
  state CrossRoad
    entry:
    LED0 = false;
    LED1 = false;
    LED2 = false;
    leftWheel = 0;
    rightWheel = 0;
    %during:
    %if (ADC14_FWD_LS >0.8* init_FWD_LEFT &&  ADC9_FWD_RS >0.8* init_FWD_RIGHT)
    %   LED1 = true;
    %else
    %    LED1 = false
    %end
    %LED_DOWN_RIGHT = false;
    %LED_DOWN_LEFT = false;
    %LED_FWD_LEFT = false;
    %LED_FWD_RIGHT = false;
    %LED_LEFT = true;
    %LED_RIGHT = true;
    %during:
    %if ADC12_LS > 0.85*init_LEFT
    %    LED2 = true;
    %else
    %   LED2 = false;
    %end
    %if ADC11_RS >0.85* init_RIGHT
    %LED0 = true;
    %else
    %    LED0 = false;
    %end
    %LED_LEFT = true;
    %LED_RIGHT = true;
    %LED_FWD_LEFT = false;
    %LED_FWD_RIGHT = false;
    %LED1 = ~LED1;
    %f ADC12_LS < 0.7* init_LEFT
    %    LED0 = true
    %end
    %if ADC11_RS < 0.7* init_RIGHT
    % LED2 = true
    %end
  state Calibration_Down1
    entry:
    LED2 = true
    LED_LEFT = false;
    LED_RIGHT = false;
    LED_FWD_LEFT = true;
    LED_FWD_RIGHT = true;
    LED_DOWN_RIGHT = true;
    LED_DOWN_LEFT = true;
    rightWheel = 75;
    leftWheel = -75;
    DOWN_R_DARK = ADC10_DOWN_RS;
    DOWN_L_DARK = ADC13_DOWN_LS;
    DOWN_R_LIGHT = ADC10_DOWN_RS;
    DOWN_L_LIGHT = ADC13_DOWN_LS;
    during:
    DOWN_R_DARK = min(DOWN_R_DARK, ADC10_DOWN_RS);
    DOWN_L_DARK = min(DOWN_L_DARK, ADC13_DOWN_LS);
    DOWN_R_LIGHT = max(DOWN_R_LIGHT, ADC10_DOWN_RS);
    DOWN_L_LIGHT = max(DOWN_L_LIGHT, ADC13_DOWN_LS);
  state WaitUntilButtonPressed6
    entry:
    LED_MOT_LEFT = false;
    LED_MOT_RIGHT = false;
    LED_FWD_LEFT = false;
    LED_FWD_RIGHT = false;
    LED_LEFT = false;
    LED_RIGHT = false;
    LED_DOWN_RIGHT = false;
    LED_DOWN_LEFT = false;
    during:
    LED1 = ~LED1;
  state Ready2
    entry:
    rightWheel = 0;
    leftWheel = 0;
    LED2 = true;
    LED0 = true;
    LED1 = true;
    maze = [
    0 1 0 0 0 1 0;
    0 1 0 1 0 1 0;
    0 0 0 1 0 0 0;
    1 1 0 0 0 1 1;
    0 0 0 1 0 0 0;
    0 1 0 1 0 1 0;
    0 0 0 0 0 0 0
    ];
    % Update flood fill matrix for a 7x7 grid
    flood = [6, 5, 4, 3, 4, 5, 6;
    5, 4, 3, 2, 3, 4, 5;
    4, 3, 2, 1, 2, 3, 4;
    3, 2, 1, 0, 1, 2, 3;  % Target cell is [4, 4] with flood value 0
    4, 3, 2, 1, 2, 3, 4;
    5, 4, 3, 2, 3, 4, 5;
    6, 5, 4, 3, 4, 5, 6];
    thresh_DOWN_RIGHT = (DOWN_R_LIGHT + DOWN_R_DARK)*0.5;
    thresh_DOWN_LEFT = (DOWN_L_LIGHT + DOWN_L_DARK)*0.5;
    SolvedAlgorithm = zeros(1, 100); % Predefine the array size
    index = 1;
  state Optimised1
    entry:
    LED0 = true;
    LED1 = true;
    LED2 = true;
    next = 0;
  state Optimised
    entry:
    LED0 = true;
    LED1 = true;
    LED2 = true;
    next = 0;
    state Done1
      entry:
      leftWheel = 0;
      rightWheel = 0;
    state Checks
      entry:
      checking = SolvedAlgorithm(index);
      exit:
      index = index+1;
    state Forward
      entry:
      leftWheel = 0;
      rightWheel = 0;
      next =1
    state TurnRight
      entry:
      leftWheel = 75;
      rightWheel = 75;
    state TurnRight2
      entry:
      leftWheel = 75;
      rightWheel = -75;
    state TurnRight3
      entry:
      leftWheel = 0;
      rightWheel = 0;
      next = 1;
    state TurnAround
      entry:
      leftWheel = 75;
      rightWheel = -75;
    state TurnAround2
      entry:
      leftWheel = 0;
      rightWheel = 0;
      next = 1;
    state TurnLeft
      entry:
      leftWheel = 75;
      rightWheel = 75;
    state TurnLeft2
      entry:
      leftWheel = -75;
      rightWheel = 75;
    state TurnLeft3
      entry:
      leftWheel = 0;
      rightWheel = 0;
      next = 1;
    Checks -> Done1 [order 5] : [checking==0]
    (default) -> Checks
    Checks -> Optimised.Forward [order 2] : [checking == S]
    Checks -> Optimised.TurnRight [order 1] : [checking == R]
    TurnRight2 -> TurnRight3 : after(1.1, sec)
    Optimised.TurnRight -> TurnRight2 : after(0.4,sec)
    Checks -> TurnAround [order 3] : [checking == B]
    TurnAround -> TurnAround2 : after (2.3,sec)
    Checks -> Optimised.TurnLeft [order 4] : [checking == L]
    Optimised.TurnLeft -> TurnLeft2 : after(0.4,sec)
    TurnLeft2 -> TurnLeft3 : after(1.2,sec)
  Turns1 -> Placeholder2 [order 2] : [SW1]
  CrossRoad -> Turns1 [order 1] : [solved == 0 && after(1,sec)]
  Turns1 -> LineFollowing [order 1] : [LED1==true]
  (default) -> WaitUntilButtonPressed10 [commented out]
  ButtonPressed8 -> Stop8 [commented out] : [ADC14_FWD_LS > init_FWD_LEFT &&  ADC9_FWD_RS > init_FWD_RIGHT]
  Calibration_Forward3 -> Calibration_Down3 [commented out] : [SW2]
  WaitUntilButtonPressed10 -> Calibration_Forward3 [commented out] : [SW1]
  Calibration_Down3 -> Ready4 [commented out] : after(5, sec)
  Ready4 -> ButtonPressed8 [commented out] : [SW1]
  Stop8 -> ButtonPressed8 [commented out] : [SW2]
  Turns -> Placeholder2 [commented out] : [SW1]
  Turns -> LineFollowing [commented out] : [LED1 ==true]
  CrossRoad -> Turns [commented out] : [solved == 0 && after(1,sec)]
  Placeholder2 -> LineFollowing : [SW2]
  LineFollowing -> Placeholder2 [order 2] : [SW1]
  ButtonPressed7 -> Stop7 [commented out] : [ADC14_FWD_LS > init_FWD_LEFT &&  ADC9_FWD_RS > init_FWD_RIGHT && SW2]
  (default) -> WaitUntilButtonPressed9 [commented out]
  Ready_To_Go2 -> ButtonPressed7 [commented out] : [SW1]
  WaitUntilButtonPressed9 -> Ready_To_Go [commented out] : [SW1]
  Side_Calibration -> Forward_Calibration [commented out] : after(4.9, sec)
      | {
      | LED_LEFT = 0;
      | LED_RIGHT = 0;
      | LED_FWD_LEFT = 1;
      | LED_FWD_RIGHT = 1;
      | }
  Forward_Calibration -> Ready_To_Go2 [commented out] : after(4.9, sec)
  Stop7 -> ButtonPressed7 [commented out] : [SW2]
  Ready_To_Go -> Side_Calibration [commented out] : [SW2]
  (default) -> WaitUntilButtonPressed6
  WaitUntilButtonPressed6 -> Calibration_Left_and_Right : [SW1]
  Calibration_Left_and_Right -> Calibration_Forward1 : [SW2]
  Calibration_Forward1 -> Calibration_Down1 : [SW1]
  Calibration_Down1 -> Ready2 : after(5, sec)
  Ready2 -> LineFollowing : [SW1]
  LineFollowing -> CrossRoad [order 1] : [ADC13_DOWN_LS < DOWN_L_DARK &&  ADC10_DOWN_RS < DOWN_R_DARK && after(1,sec)]
  CrossRoad -> LineFollowing [order 2] : [SW2]
  Optimised -> LineFollowing : [next==1]
  CrossRoad -> Optimised [order 3] : [solved == 1 && after(1,sec)]
  data: ADC14_FWD_LS input; ADC13_DOWN_LS input; ADC12_LS input; ADC11_RS input; ADC10_DOWN_RS input; ADC9_FWD_RS input; ADC8_MOT_RS input; leftWheel output; rightWheel output; LED_FWD_LEFT output; LED_DOWN_LEFT output; LED1 output =false; LED2 output =false; LED_LEFT output; LED_RIGHT output; LED_DOWN_RIGHT output; LED_FWD_RIGHT output; SW2 input; LED0 output =false; SW1 input; init_FWD_RIGHT local; init_FWD_LEFT local; DOWN_L_LIGHT local; thresh_DOWN_LEFT local; normal_speed_RIGHT local; DOWN_R_DARK local; DOWN_L_DARK local; thresh_DOWN_RIGHT local; DOWN_R_LIGHT local; normal_speed_LEFT local; avg_FWD_LEFT local; counter local; avg_FWD_RIGHT local; sum_FWD_LEFT local uint16; sum_FWD_RIGHT local uint16; avg_LEFT local; avg_RIGHT local; init_LEFT local; init_RIGHT local; sum_LEFT local uint16; sum_RIGHT local uint16; timer local; dark_val_l local; fwd_count local; light_val_r local; dark_val_r local; light_val_l local; lr_count local; motor_speed_left local; motor_speed_right local; thresh_LEFT local; thresh_RIGHT local; thresh_down_l local; thresh_down_r local; averageDown local; averageFront local; crossThreshold local; frontThreshold local; LED_MOT_LEFT local; LED_MOT_RIGHT local; flag local; counter2 local; R local; SolvedAlgorithm local; B local; checking local; index local; L local; next local; solved local; S local; flood local; ADC15_MOT_LS local; maze local; stop local
